simulink model "LAb4_4"  (R2024b)
settings: Solver=VariableStepAuto  StartTime=0.0  StopTime=inf  RelTol=1e-3
libraries: commfilt2 x2, commdigbbndam3 x2, commchan3 x1, commsink2 x1, dspvision x1, simulink x1
settings Model: Creator=Jose  LastModifiedBy=Jose

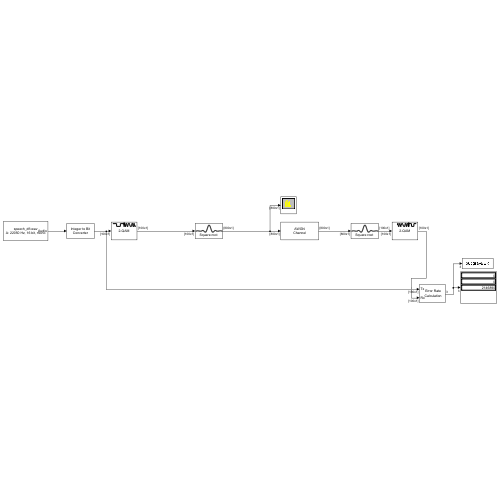
[thumbnail: Simulink's stored preview of the top-level diagram]
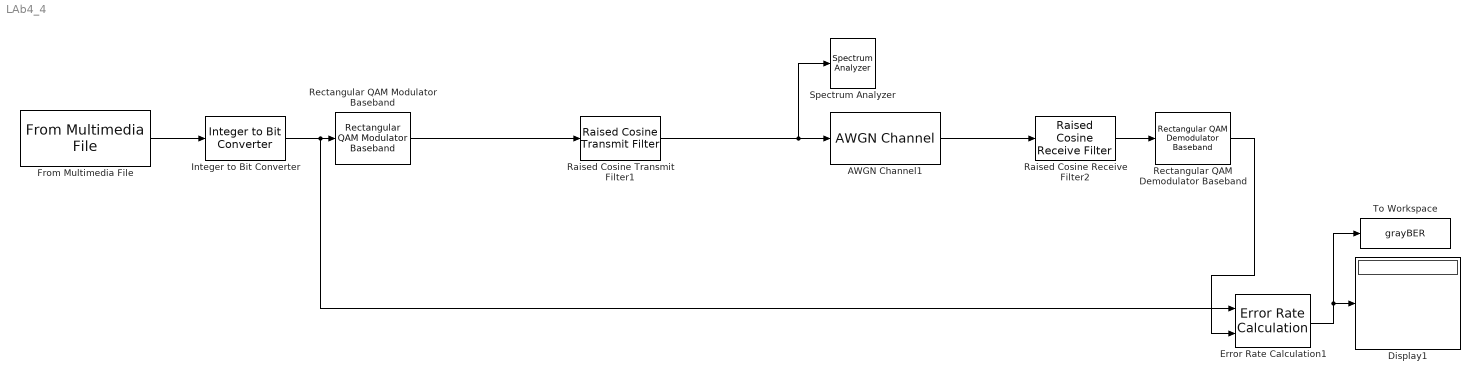
== system LAb4_4 ==
  AWGN Channel1 : commchan3/AWGN Channel  LegacyMode=off  NoiseMethod="Signal to noise ratio  (Eb/No)"  noiseMode="Signal to noise ratio  (SNR)"  EbNo=10  EsNo=10  SNR=10  BitsPerSymbol=1  SignalPower=1/(2*8)  SamplesPerSymbol=8  SymbolPeriod=1  VarianceSource=Parameter  Variance=1  RandomStream=mt19937ar with seed  Seed=67  SimulateUsing=Code generation
  Display1 : Display
  Error Rate Calculation1 : commsink2/Error Rate Calculation  N=10  st_delay=0  cp_mode=Entire frame  subframe=[]  PMode=Port  WsName=ErrorVec  RsMode2=off  stop=off  numErr=100  maxBits=1e6
      settings: LibrarySourceBlock=|
      | commhdlsink/Error Rate
      | Calculation
  From Multimedia File : dspvision/From Multimedia File  inputFilename=C:\Program Files\MATLAB\R2024b\toolbox\dsp\dsp\samples\speech_dft.wav  readRange=[1 Inf]  loop=on  numPlays=inf  outputStreams=Audio only  videoDataType=single  audioDataType=int16  inheritSampleTime=on  userDefinedSampleTime=1/30  noAudioOutput=off  isIntensityVideo=off  fourcc=RGB  colorVideoFormat=Separate color signals  outputEOF=off  dataOrg=Column-major  audioFrameSize=1024  computeAudioFrameSize=off  outSamplingMode=Sample based
  Integer to Bit Converter : simulink/Logic and Bit Operations/Integer to Bit Converter  nbits=16  signedInputValues=Signed  bitOrder=MSB first  outDtype=double
      settings: LibrarySourceBlock=|
      | commutil2/Integer to Bit
      | Converter
  Raised Cosine Receive Filter2 : commfilt2/Raised Cosine Receive Filter  filtType=Square root  R=1  filtSpan=10  N=8  downFactor=8  downOffset=0  filterGain=2  InputProcessing=Columns as channels (frame based)  RateOptions=Enforce single-rate processing  framing=Mute  checkCoeff=off  variableName=rcRxFilt2  currentFiltSpan=10  D=5  inputOffset=0  sampMode=Mute  saveAsFlag=0  rateMode=Downsampling  checkGain=Normalized  launchFVT=on  roundingMode=Floor  overflowMode=off  coeffDataTypeStr=Inherit: Same word length as input  coeffMin=[]  coeffMax=[]  coeffLastDataTypeStr=Inherit: Same word length as input  accumDataTypeStr=Inherit: Same as product output  accumLastDataTypeStr=Inherit: Same as product output  outputDataTypeStr=Inherit: Same as accumulator  outputMin=[]  outputMax=[]  outputLastDataTypeStr=Inherit: Same as accumulator
      settings: LibrarySourceBlock=|
      | commhdlfilt/Raised Cosine
      | Receive Filter
  Raised Cosine Transmit Filter1 : commfilt2/Raised Cosine Transmit Filter  filtType=Square root  R=1  filtSpan=10  N=8  filterGain=1  InputProcessing=Columns as channels (frame based)  RateOptions=Enforce single-rate processing  framing=Mute  checkCoeff=off  variableName=rcTxFilt1  checkGain=Normalized  sampMode=Mute  saveAsFlag=0  currentFiltSpan=10  D=5  launchFVT=on  roundingMode=Floor  overflowMode=off  coeffDataTypeStr=Inherit: Same word length as input  coeffMin=[]  coeffMax=[]  coeffLastDataTypeStr=Inherit: Same word length as input  outputDataTypeStr=Inherit: Same as accumulator  outputMin=[]  outputMax=[]  outputLastDataTypeStr=Inherit: Same as accumulator
      settings: LibrarySourceBlock=|
      | commhdlfilt/Raised Cosine
      | Transmit Filter
  Rectangular QAM Demodulator Baseband : commdigbbndam3/Rectangular QAM Demodulator Baseband  M=2  OutType=Bit  DecType=Hard decision  VarSource=Dialog  Variance=1  Dec=Gray  Mapping=[0:15]  PowType=Average Power  MinDist=2  AvgPow=1  PeakPow=1  Ph=0  outDtype1=Inherit via internal rule  outDtype2=Inherit via internal rule  derotateFactorWordLen=16  derotateFactorDataTypeStr=Inherit: Same word length as input  derotateFactorLastDataTypeStr=Inherit: Same word length as input  denormFactorWordLen=16  denormFactorDataTypeStr=Inherit: Same word length as input  denormFactorLastDataTypeStr=Inherit: Same word length as input  prodOutWordLen=32  prodOutOverflowMode=Wrap  prodOutRoundingMode=Floor  prodOutOvFlMode=off  prodOutOvFlModeLastStrValue=off  sumWordLen=32
      settings: LibrarySourceBlock=|
      | commhdldigbbndam/Rectangular QAM
      | Demodulator
      | Baseband
  Rectangular QAM Modulator Baseband : commdigbbndam3/Rectangular QAM Modulator Baseband  M=2  InType=Bit  Enc=Gray  Mapping=[0:15]  PowType=Min. distance between symbols  MinDist=2  AvgPow=1  PeakPow=1  Ph=0  outDtype=double  outWordLen=16  outUDDataType=sfix(16)  outFracLenMode=Best precision  outFracLen=15  outDataTypeStr=double  outLastDataTypeStr=double
      settings: LibrarySourceBlock=|
      | commhdldigbbndam/Rectangular QAM
      | Modulator
      | Baseband
  Spectrum Analyzer : SpectrumAnalyzer  WindowPosition=[368.000000,182.000000,800.000000,498.000000,]  ScopeFrameLocation=window  WindowInvariantSamplesPerUpdate=on  Span=8000000.000000001  StartFrequency=-4000000.0000000005  StopFrequency=4000000.0000000005  YLimits=[-104.50099361,14.46877151]
  To Workspace : ToWorkspace  VariableName=grayBER  SampleTime=-1
      settings: MaxDataPoints=2  Save2DSignal=2-D array (concatenate along first dimension)
  wires:
  Rectangular QAM Demodulator Baseband/1 -> Error Rate Calculation1/2
  Integer to Bit Converter/1 -> Rectangular QAM Modulator Baseband/1, Error Rate Calculation1/1
  Rectangular QAM Modulator Baseband/1 -> Raised Cosine Transmit Filter1/1
  Error Rate Calculation1/1 -> To Workspace/1, Display1/1
  Raised Cosine Receive Filter2/1 -> Rectangular QAM Demodulator Baseband/1
  Raised Cosine Transmit Filter1/1 -> Spectrum Analyzer/1, AWGN Channel1/1
  AWGN Channel1/1 -> Raised Cosine Receive Filter2/1
  From Multimedia File/1 -> Integer to Bit Converter/1
